simulink model "Zad2"  (Simulink 8.6)
settings: Solver=ode45  StartTime=0.0  StopTime=t_sim  RelTol=1e-3
values from neighbouring files (symbols this model uses):
  ICX = -0.2    [zadatak1.m]    (also in zadatak2.m = 2; zadatak4.m = 0.4)
  ICY = -0.6    [zadatak1.m]    (also in zadatak2.m = 4; zadatak4.m = 1)
libraries: fuzblock x1
settings Model: Creator=Domagoj  LastModifiedBy=Branko
settings DebuggingCC: SolverPrmCheckMsg=none  FcnCallInpInsideContextMsg=UseLocalSettings

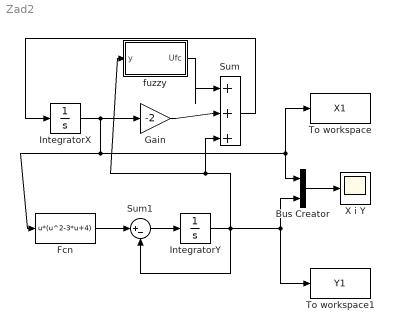
== system Zad2 ==
  Bus Creator : BusCreator  Inputs=2
  Fcn : Fcn  Expr=u*(u^2-3*u+4)
  Gain : Gain  Gain=-2
  IntegratorX : Integrator  InitialCondition=ICX  UpperSaturationLimit=10000
  IntegratorY : Integrator  InitialCondition=ICY  UpperSaturationLimit=10000
  Sum : Sum  Inputs=|+++
  Sum1 : Sum  Inputs=|+-
  To workspace : ToWorkspace  VariableName=X1  SampleTime=-1
  To workspace1 : ToWorkspace  VariableName=Y1  SampleTime=-1
  X i Y : Scope
  fuzzy : Subsystem
  wires:
  Sum/1 -> IntegratorX/1
  IntegratorY/1 -> To workspace1/1, Bus Creator/2, Sum1/2, Sum/3, fuzzy/1(y)
  Bus Creator/1 -> X i Y/1
  Fcn/1 -> Sum1/1
  Sum1/1 -> IntegratorY/1
  Gain/1 -> Sum/2
  IntegratorX/1 -> Gain/1, Fcn/1, Bus Creator/1, To workspace/1
  fuzzy/1(Ufc) -> Sum/1

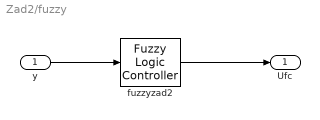
== system Zad2/fuzzy ==
  y : Inport
  fuzzyzad2 : fuzblock/Fuzzy Logic  Controller  fis=fuzzyPI1
  Ufc : Outport
  wires:
  y/1 -> fuzzyzad2/1
  fuzzyzad2/1 -> Ufc/1
